simulink model "bench_loco"  (R2024b)
settings: Solver=daessc  StartTime=0.0  StopTime=120  MaxStep=1e-2  RelTol=1e-3
values from neighbouring files (symbols this model uses):
  PN = evalin('base','PN')    [run_bench_string_heat.m]
libraries: loco_native_lib x13, fl_lib x4, nesl_utility x3
settings Model: Creator=BillBeverley  LastModifiedBy=BillBeverley

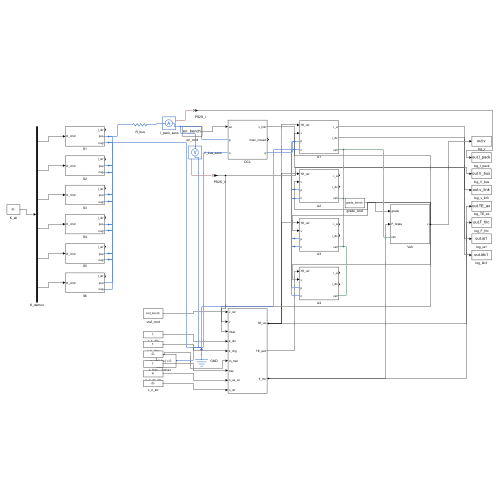
[thumbnail: Simulink's stored preview of the top-level diagram]
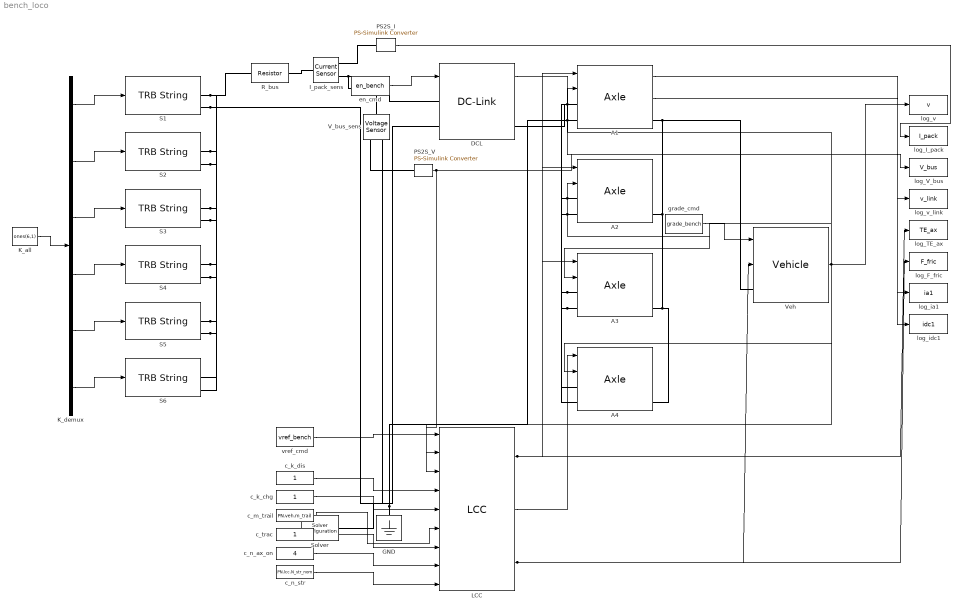
== system bench_loco ==
  A{1..4} (4 alike) : loco_native_lib/Axle  SystemSampleTime=-1  VariantActivationTime=update diagram  AllowFlexibleInterface=on  Latency=0  AutoFrameSizeCalculation=off
  DCL : loco_native_lib/DC-Link  SystemSampleTime=-1  VariantActivationTime=update diagram  AllowFlexibleInterface=on  Latency=0  AutoFrameSizeCalculation=off
  GND : fl_lib/Electrical/Electrical Elements/Electrical Reference
  I_pack_sens : fl_lib/Electrical/Electrical Sensors/Current Sensor
  K_all : Constant  Value=ones(6,1)
  K_demux : Demux  Outputs=6
  LCC : loco_native_lib/LCC  L=PN.lcc
  PS2S_I : nesl_utility/PS-Simulink Converter  PhysicalDomain=network_engine_domain  SubClassName=ps_output  LeftPortType=input  RightPortType=output  PseudoPeriodic=off  Frequencies=[]  VectorFormat=inherit  Unit=A  AffineConversion=off
  PS2S_V : nesl_utility/PS-Simulink Converter  PhysicalDomain=network_engine_domain  SubClassName=ps_output  LeftPortType=input  RightPortType=output  PseudoPeriodic=off  Frequencies=[]  VectorFormat=inherit  Unit=V  AffineConversion=off
  R_bus : fl_lib/Electrical/Electrical Elements/Resistor  R=PN.bus.R Ohm  i_specify=off  i_priority=None  i=0 A  i_nominal_specify=off  i_nominal_value=1  i_nominal_unit=A  v_specify=off  v_priority=None  v=0 V  v_nominal_specify=off  v_nominal_value=1  v_nominal_unit=V
  S{1..6} (6 alike) : loco_native_lib/TRB String  SystemSampleTime=-1  VariantActivationTime=update diagram  AllowFlexibleInterface=on  Latency=0  AutoFrameSizeCalculation=off
  Solver : nesl_utility/Solver Configuration  PhysicalDomain=network_engine_domain  SubClassName=solver  LeftPortType=input  RightPortType=generic  Tones=[]  Harmonics=[]  SimulateNoise=off  Profile=off  UseLocalSampling=off  EnableSwitchedLinearOptims=on  FrequencyDomain=off  UseCCode=off  RelTol=0.001  AbsTol=0.001  MinStep=1e-09  ToWorkspace=off  RevertToSquareIcSolve=off  NumHomotopyIterations=100  PhasorMode=off  PhasorModeNumHarmonics=1  ConsistencySolver=NEWTON_XTOL_AFTER_FTOL  IndexReductionMethod=DerivativeReplacement  DoDC=off  ResidualTolerance=1e-09  ConsistencyTolSource=GLOBAL  ConsistencyAbsTol=0.001  ConsistencyRelTol=0.001  ConsistencyTolFactor=0.001  UseLocalSolver=off  LocalSolverChoice=NE_BACKWARD_EULER_ADVANCER  ResolveIndetEquations=on  FunctionEvalNumThread=1  LocalSolverSampleTime=0.001  DoFixedCost=off  MaxNonlinIter=3  MaxModeIter=2  ComputeImpulses=off  ImpulseIterations=2  LinearAlgebra=auto  LinearAlgebraNumThread=0  EquationFormulation=NE_TIME_EF  DelaysMemoryBudget=1024  AutomaticFiltering=on  FilteringTimeConstant=0.001  PartitionStorageMethod=AS_NEEDED  PartitionMemoryBudget=1024  PartitionMethod=ROBUST  MultibodyUseLocalSolver=off  MultibodyLocalSolverChoice=ODE1  MultibodyLocalSolverSampleTime=0.001
  V_bus_sens : fl_lib/Electrical/Electrical Sensors/Voltage Sensor
  Veh : loco_native_lib/Vehicle  SystemSampleTime=-1  VariantActivationTime=update diagram  AllowFlexibleInterface=on  Latency=0  AutoFrameSizeCalculation=off
  c_k_chg : Constant
  c_k_dis : Constant
  c_m_trail : Constant  Value=PN.veh.m_trail
  c_n_ax_on : Constant  Value=4
  c_n_str : Constant  Value=PN.lcc.N_str_nom
  c_trac : Constant
  en_cmd : FromWorkspace  VariableName=en_bench
  grade_cmd : FromWorkspace  VariableName=grade_bench
  log_F_fric : ToWorkspace  VariableName=F_fric  SaveFormat=Timeseries  SampleTime=-1
  log_I_pack : ToWorkspace  VariableName=I_pack  SaveFormat=Timeseries  SampleTime=-1
  log_TE_ax : ToWorkspace  VariableName=TE_ax  SaveFormat=Timeseries  SampleTime=-1
  log_V_bus : ToWorkspace  VariableName=V_bus  SaveFormat=Timeseries  SampleTime=-1
  log_ia1 : ToWorkspace  VariableName=ia1  SaveFormat=Timeseries  SampleTime=-1
  log_idc1 : ToWorkspace  VariableName=idc1  SaveFormat=Timeseries  SampleTime=-1
  log_v : ToWorkspace  VariableName=v  SaveFormat=Timeseries  SampleTime=-1
  log_v_link : ToWorkspace  VariableName=v_link  SaveFormat=Timeseries  SampleTime=-1
  vref_cmd : FromWorkspace  VariableName=vref_bench
  wires:
  Veh/1 -> log_v/1, LCC/2, A1/2, A2/2, A3/2, A4/2
  PS2S_I/1 -> log_I_pack/1
  PS2S_V/1 -> log_V_bus/1, LCC/3
  DCL/1 -> log_v_link/1
  LCC/1 -> log_TE_ax/1, A1/1, A2/1, A3/1
  LCC/3 -> log_F_fric/1, Veh/2
  A1/1 -> log_ia1/1
  A1/2 -> log_idc1/1
  K_all/1 -> K_demux/1
  en_cmd/1 -> DCL/1
  vref_cmd/1 -> LCC/1
  c_k_dis/1 -> LCC/4
  c_k_chg/1 -> LCC/5
  c_m_trail/1 -> LCC/6
  c_trac/1 -> LCC/7
  c_n_ax_on/1 -> LCC/8
  c_n_str/1 -> LCC/9
  LCC/2 -> A4/1
  grade_cmd/1 -> Veh/1
  K_demux/1 -> S1/1
  K_demux/2 -> S2/1
  K_demux/3 -> S3/1
  K_demux/4 -> S4/1
  K_demux/5 -> S5/1
  K_demux/6 -> S6/1
  connections:
  R_bus/LConn1 -- S1/RConn1 -- S2/RConn1 -- S3/RConn1 -- S4/RConn1 -- S5/RConn1 -- S6/RConn1
  R_bus/RConn1 -- I_pack_sens/LConn1
  DCL/LConn1 -- I_pack_sens/RConn2 -- V_bus_sens/LConn1
  V_bus_sens/RConn2 -- S1/RConn2 -- S2/RConn2 -- S3/RConn2 -- S4/RConn2 -- S5/RConn2 -- S6/RConn2 -- DCL/LConn2 -- Solver/RConn1 -- GND/LConn1 -- A1/LConn2 -- A2/LConn2 -- A3/LConn2 -- A4/LConn2
  I_pack_sens/RConn1 -- PS2S_I/LConn1
  V_bus_sens/RConn1 -- PS2S_V/LConn1
  A1/LConn1 -- DCL/RConn1 -- A2/LConn1 -- A3/LConn1 -- A4/LConn1
  Veh/LConn1 -- A1/RConn1 -- A2/RConn1 -- A3/RConn1 -- A4/RConn1
